simulink model "questao2a"  (Simulink 7.1)
settings: Solver=ode45  StartTime=0.0  StopTime=10.0  RelTol=1e-3
settings Model: Creator=ALUNO  LastModifiedBy=ALUNO

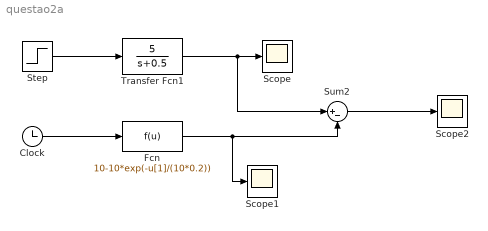
== system questao2a ==
  Clock : Clock
      settings: Decimation=10
  Fcn : Fcn  Expr=10-10*exp(-u[1]/(10*0.2))
  Scope : Scope
  Scope1 : Scope
  Scope2 : Scope
      settings: SaveName=ScopeData2
  Step : Step  Time=0  SampleTime=0
  Sum2 : Sum  Inputs=|+-  OutDataType=sfix(16)  OutScaling=2^0
  Transfer Fcn1 : TransferFcn  Numerator=[5]  Denominator=[1 0.5]
  wires:
  Step/1 -> Transfer Fcn1/1
  Transfer Fcn1/1 -> Scope/1, Sum2/1
  Fcn/1 -> Scope1/1, Sum2/2
  Clock/1 -> Fcn/1
  Sum2/1 -> Scope2/1
